simulink model "adc16_dbf_4fft"  (R2013a)
settings: Solver=ode45  StartTime=0.0  StopTime=2050  RelTol=1e-3
undefined symbols (not defined in the file): pfb_coeff_gen_calc
libraries: xbsIndex_r4 x1713, casper_library_misc x294, casper_library_delays x48, casper_library_pfbs x16, simulink x16, xps_library x1
(part 2 of 21)

== system adc16_dbf_4fft/gateway10 ==
  data[4] : Inport
  Bus Creator : BusCreator
  Bus Selector : BusSelector  OutputSignals=signal1,signal2,signal3,signal4
  Gateway Out{,1..3} (4 alike) : xbsIndex_r4/Gateway Out  inherit_from_input=off  hdl_port=on  timing_constraint=None  locs_specified=off  LOCs={}  UseAsDAC=off  DACChannel='1'  block_type=gatewayout
  to_scope : Outport
  wires:
  data[4]/1 -> Bus Selector/1
  Bus Selector/4 -> Gateway Out3/1  "<signal4>"
  Bus Selector/2 -> Gateway Out1/1  "<signal2>"
  Bus Selector/1 -> Gateway Out/1  "<signal1>"
  Bus Selector/3 -> Gateway Out2/1  "<signal3>"
  Bus Creator/1 -> to_scope/1
  Gateway Out/1 -> Bus Creator/1
  Gateway Out1/1 -> Bus Creator/2
  Gateway Out2/1 -> Bus Creator/3
  Gateway Out3/1 -> Bus Creator/4

== system adc16_dbf_4fft/gateway11 ==
  data[4] : Inport
  Bus Creator : BusCreator
  Bus Selector : BusSelector  OutputSignals=signal1,signal2,signal3,signal4
  Gateway Out{,1..3} (4 alike) : xbsIndex_r4/Gateway Out  inherit_from_input=off  hdl_port=on  timing_constraint=None  locs_specified=off  LOCs={}  UseAsDAC=off  DACChannel='1'  block_type=gatewayout
  to_scope : Outport
  wires:
  Gateway Out3/1 -> Bus Creator/4
  Gateway Out2/1 -> Bus Creator/3
  Gateway Out1/1 -> Bus Creator/2
  Gateway Out/1 -> Bus Creator/1
  Bus Creator/1 -> to_scope/1
  Bus Selector/3 -> Gateway Out2/1  "<signal3>"
  Bus Selector/1 -> Gateway Out/1  "<signal1>"
  Bus Selector/2 -> Gateway Out1/1  "<signal2>"
  Bus Selector/4 -> Gateway Out3/1  "<signal4>"
  data[4]/1 -> Bus Selector/1

== system adc16_dbf_4fft/gateway12 ==
  data[4] : Inport
  Bus Creator : BusCreator
  Bus Selector : BusSelector  OutputSignals=signal1,signal2,signal3,signal4
  Gateway Out{,1..3} (4 alike) : xbsIndex_r4/Gateway Out  inherit_from_input=off  hdl_port=on  timing_constraint=None  locs_specified=off  LOCs={}  UseAsDAC=off  DACChannel='1'  block_type=gatewayout
  to_scope : Outport
  wires:
  Gateway Out3/1 -> Bus Creator/4
  Gateway Out2/1 -> Bus Creator/3
  Gateway Out1/1 -> Bus Creator/2
  Gateway Out/1 -> Bus Creator/1
  Bus Creator/1 -> to_scope/1
  Bus Selector/3 -> Gateway Out2/1  "<signal3>"
  Bus Selector/1 -> Gateway Out/1  "<signal1>"
  Bus Selector/2 -> Gateway Out1/1  "<signal2>"
  Bus Selector/4 -> Gateway Out3/1  "<signal4>"
  data[4]/1 -> Bus Selector/1

== system adc16_dbf_4fft/gateway13 ==
  data[4] : Inport
  Bus Creator : BusCreator
  Bus Selector : BusSelector  OutputSignals=signal1,signal2,signal3,signal4
  Gateway Out{,1..3} (4 alike) : xbsIndex_r4/Gateway Out  inherit_from_input=off  hdl_port=on  timing_constraint=None  locs_specified=off  LOCs={}  UseAsDAC=off  DACChannel='1'  block_type=gatewayout
  to_scope : Outport
  wires:
  data[4]/1 -> Bus Selector/1
  Bus Selector/4 -> Gateway Out3/1  "<signal4>"
  Bus Selector/2 -> Gateway Out1/1  "<signal2>"
  Bus Selector/1 -> Gateway Out/1  "<signal1>"
  Bus Selector/3 -> Gateway Out2/1  "<signal3>"
  Bus Creator/1 -> to_scope/1
  Gateway Out/1 -> Bus Creator/1
  Gateway Out1/1 -> Bus Creator/2
  Gateway Out2/1 -> Bus Creator/3
  Gateway Out3/1 -> Bus Creator/4

== system adc16_dbf_4fft/gateway14 ==
  data[4] : Inport
  Bus Creator : BusCreator
  Bus Selector : BusSelector  OutputSignals=signal1,signal2,signal3,signal4
  Gateway Out{,1..3} (4 alike) : xbsIndex_r4/Gateway Out  inherit_from_input=off  hdl_port=on  timing_constraint=None  locs_specified=off  LOCs={}  UseAsDAC=off  DACChannel='1'  block_type=gatewayout
  to_scope : Outport
  wires:
  Gateway Out3/1 -> Bus Creator/4
  Gateway Out2/1 -> Bus Creator/3
  Gateway Out1/1 -> Bus Creator/2
  Gateway Out/1 -> Bus Creator/1
  Bus Creator/1 -> to_scope/1
  Bus Selector/3 -> Gateway Out2/1  "<signal3>"
  Bus Selector/1 -> Gateway Out/1  "<signal1>"
  Bus Selector/2 -> Gateway Out1/1  "<signal2>"
  Bus Selector/4 -> Gateway Out3/1  "<signal4>"
  data[4]/1 -> Bus Selector/1

== system adc16_dbf_4fft/gateway15 ==
  data[4] : Inport
  Bus Creator : BusCreator
  Bus Selector : BusSelector  OutputSignals=signal1,signal2,signal3,signal4
  Gateway Out{,1..3} (4 alike) : xbsIndex_r4/Gateway Out  inherit_from_input=off  hdl_port=on  timing_constraint=None  locs_specified=off  LOCs={}  UseAsDAC=off  DACChannel='1'  block_type=gatewayout
  to_scope : Outport
  wires:
  data[4]/1 -> Bus Selector/1
  Bus Selector/4 -> Gateway Out3/1  "<signal4>"
  Bus Selector/2 -> Gateway Out1/1  "<signal2>"
  Bus Selector/1 -> Gateway Out/1  "<signal1>"
  Bus Selector/3 -> Gateway Out2/1  "<signal3>"
  Bus Creator/1 -> to_scope/1
  Gateway Out/1 -> Bus Creator/1
  Gateway Out1/1 -> Bus Creator/2
  Gateway Out2/1 -> Bus Creator/3
  Gateway Out3/1 -> Bus Creator/4

== system adc16_dbf_4fft/gateway16 ==
  data[4] : Inport
  Bus Creator : BusCreator
  Bus Selector : BusSelector  OutputSignals=signal1,signal2,signal3,signal4
  Gateway Out{,1..3} (4 alike) : xbsIndex_r4/Gateway Out  inherit_from_input=off  hdl_port=on  timing_constraint=None  locs_specified=off  LOCs={}  UseAsDAC=off  DACChannel='1'  block_type=gatewayout
  to_scope : Outport
  wires:
  Gateway Out3/1 -> Bus Creator/4
  Gateway Out2/1 -> Bus Creator/3
  Gateway Out1/1 -> Bus Creator/2
  Gateway Out/1 -> Bus Creator/1
  Bus Creator/1 -> to_scope/1
  Bus Selector/3 -> Gateway Out2/1  "<signal3>"
  Bus Selector/1 -> Gateway Out/1  "<signal1>"
  Bus Selector/2 -> Gateway Out1/1  "<signal2>"
  Bus Selector/4 -> Gateway Out3/1  "<signal4>"
  data[4]/1 -> Bus Selector/1

== system adc16_dbf_4fft/gateway2 ==
  data[4] : Inport
  Bus Creator : BusCreator
  Bus Selector : BusSelector  OutputSignals=signal1,signal2,signal3,signal4
  Gateway Out{,1..3} (4 alike) : xbsIndex_r4/Gateway Out  inherit_from_input=off  hdl_port=on  timing_constraint=None  locs_specified=off  LOCs={}  UseAsDAC=off  DACChannel='1'  block_type=gatewayout
  to_scope : Outport
  wires:
  data[4]/1 -> Bus Selector/1
  Bus Selector/4 -> Gateway Out3/1  "<signal4>"
  Bus Selector/2 -> Gateway Out1/1  "<signal2>"
  Bus Selector/1 -> Gateway Out/1  "<signal1>"
  Bus Selector/3 -> Gateway Out2/1  "<signal3>"
  Bus Creator/1 -> to_scope/1
  Gateway Out/1 -> Bus Creator/1
  Gateway Out1/1 -> Bus Creator/2
  Gateway Out2/1 -> Bus Creator/3
  Gateway Out3/1 -> Bus Creator/4

== system adc16_dbf_4fft/gateway3 ==
  data[4] : Inport
  Bus Creator : BusCreator
  Bus Selector : BusSelector  OutputSignals=signal1,signal2,signal3,signal4
  Gateway Out{,1..3} (4 alike) : xbsIndex_r4/Gateway Out  inherit_from_input=off  hdl_port=on  timing_constraint=None  locs_specified=off  LOCs={}  UseAsDAC=off  DACChannel='1'  block_type=gatewayout
  to_scope : Outport
  wires:
  data[4]/1 -> Bus Selector/1
  Bus Selector/4 -> Gateway Out3/1  "<signal4>"
  Bus Selector/2 -> Gateway Out1/1  "<signal2>"
  Bus Selector/1 -> Gateway Out/1  "<signal1>"
  Bus Selector/3 -> Gateway Out2/1  "<signal3>"
  Bus Creator/1 -> to_scope/1
  Gateway Out/1 -> Bus Creator/1
  Gateway Out1/1 -> Bus Creator/2
  Gateway Out2/1 -> Bus Creator/3
  Gateway Out3/1 -> Bus Creator/4

== system adc16_dbf_4fft/gateway4 ==
  data[4] : Inport
  Bus Creator : BusCreator
  Bus Selector : BusSelector  OutputSignals=signal1,signal2,signal3,signal4
  Gateway Out{,1..3} (4 alike) : xbsIndex_r4/Gateway Out  inherit_from_input=off  hdl_port=on  timing_constraint=None  locs_specified=off  LOCs={}  UseAsDAC=off  DACChannel='1'  block_type=gatewayout
  to_scope : Outport
  wires:
  Gateway Out3/1 -> Bus Creator/4
  Gateway Out2/1 -> Bus Creator/3
  Gateway Out1/1 -> Bus Creator/2
  Gateway Out/1 -> Bus Creator/1
  Bus Creator/1 -> to_scope/1
  Bus Selector/3 -> Gateway Out2/1  "<signal3>"
  Bus Selector/1 -> Gateway Out/1  "<signal1>"
  Bus Selector/2 -> Gateway Out1/1  "<signal2>"
  Bus Selector/4 -> Gateway Out3/1  "<signal4>"
  data[4]/1 -> Bus Selector/1

== system adc16_dbf_4fft/gateway5 ==
  data[4] : Inport
  Bus Creator : BusCreator
  Bus Selector : BusSelector  OutputSignals=signal1,signal2,signal3,signal4
  Gateway Out{,1..3} (4 alike) : xbsIndex_r4/Gateway Out  inherit_from_input=off  hdl_port=on  timing_constraint=None  locs_specified=off  LOCs={}  UseAsDAC=off  DACChannel='1'  block_type=gatewayout
  to_scope : Outport
  wires:
  data[4]/1 -> Bus Selector/1
  Bus Selector/4 -> Gateway Out3/1  "<signal4>"
  Bus Selector/2 -> Gateway Out1/1  "<signal2>"
  Bus Selector/1 -> Gateway Out/1  "<signal1>"
  Bus Selector/3 -> Gateway Out2/1  "<signal3>"
  Bus Creator/1 -> to_scope/1
  Gateway Out/1 -> Bus Creator/1
  Gateway Out1/1 -> Bus Creator/2
  Gateway Out2/1 -> Bus Creator/3
  Gateway Out3/1 -> Bus Creator/4

== system adc16_dbf_4fft/gateway6 ==
  data[4] : Inport
  Bus Creator : BusCreator
  Bus Selector : BusSelector  OutputSignals=signal1,signal2,signal3,signal4
  Gateway Out{,1..3} (4 alike) : xbsIndex_r4/Gateway Out  inherit_from_input=off  hdl_port=on  timing_constraint=None  locs_specified=off  LOCs={}  UseAsDAC=off  DACChannel='1'  block_type=gatewayout
  to_scope : Outport
  wires:
  data[4]/1 -> Bus Selector/1
  Bus Selector/4 -> Gateway Out3/1  "<signal4>"
  Bus Selector/2 -> Gateway Out1/1  "<signal2>"
  Bus Selector/1 -> Gateway Out/1  "<signal1>"
  Bus Selector/3 -> Gateway Out2/1  "<signal3>"
  Bus Creator/1 -> to_scope/1
  Gateway Out/1 -> Bus Creator/1
  Gateway Out1/1 -> Bus Creator/2
  Gateway Out2/1 -> Bus Creator/3
  Gateway Out3/1 -> Bus Creator/4

== system adc16_dbf_4fft/gateway7 ==
  data[4] : Inport
  Bus Creator : BusCreator
  Bus Selector : BusSelector  OutputSignals=signal1,signal2,signal3,signal4
  Gateway Out{,1..3} (4 alike) : xbsIndex_r4/Gateway Out  inherit_from_input=off  hdl_port=on  timing_constraint=None  locs_specified=off  LOCs={}  UseAsDAC=off  DACChannel='1'  block_type=gatewayout
  to_scope : Outport
  wires:
  Gateway Out3/1 -> Bus Creator/4
  Gateway Out2/1 -> Bus Creator/3
  Gateway Out1/1 -> Bus Creator/2
  Gateway Out/1 -> Bus Creator/1
  Bus Creator/1 -> to_scope/1
  Bus Selector/3 -> Gateway Out2/1  "<signal3>"
  Bus Selector/1 -> Gateway Out/1  "<signal1>"
  Bus Selector/2 -> Gateway Out1/1  "<signal2>"
  Bus Selector/4 -> Gateway Out3/1  "<signal4>"
  data[4]/1 -> Bus Selector/1

== system adc16_dbf_4fft/gateway8 ==
  data[4] : Inport
  Bus Creator : BusCreator
  Bus Selector : BusSelector  OutputSignals=signal1,signal2,signal3,signal4
  Gateway Out{,1..3} (4 alike) : xbsIndex_r4/Gateway Out  inherit_from_input=off  hdl_port=on  timing_constraint=None  locs_specified=off  LOCs={}  UseAsDAC=off  DACChannel='1'  block_type=gatewayout
  to_scope : Outport
  wires:
  Gateway Out3/1 -> Bus Creator/4
  Gateway Out2/1 -> Bus Creator/3
  Gateway Out1/1 -> Bus Creator/2
  Gateway Out/1 -> Bus Creator/1
  Bus Creator/1 -> to_scope/1
  Bus Selector/3 -> Gateway Out2/1  "<signal3>"
  Bus Selector/1 -> Gateway Out/1  "<signal1>"
  Bus Selector/2 -> Gateway Out1/1  "<signal2>"
  Bus Selector/4 -> Gateway Out3/1  "<signal4>"
  data[4]/1 -> Bus Selector/1

== system adc16_dbf_4fft/gateway9 ==
  data[4] : Inport
  Bus Creator : BusCreator
  Bus Selector : BusSelector  OutputSignals=signal1,signal2,signal3,signal4
  Gateway Out{,1..3} (4 alike) : xbsIndex_r4/Gateway Out  inherit_from_input=off  hdl_port=on  timing_constraint=None  locs_specified=off  LOCs={}  UseAsDAC=off  DACChannel='1'  block_type=gatewayout
  to_scope : Outport
  wires:
  data[4]/1 -> Bus Selector/1
  Bus Selector/4 -> Gateway Out3/1  "<signal4>"
  Bus Selector/2 -> Gateway Out1/1  "<signal2>"
  Bus Selector/1 -> Gateway Out/1  "<signal1>"
  Bus Selector/3 -> Gateway Out2/1  "<signal3>"
  Bus Creator/1 -> to_scope/1
  Gateway Out/1 -> Bus Creator/1
  Gateway Out1/1 -> Bus Creator/2
  Gateway Out2/1 -> Bus Creator/3
  Gateway Out3/1 -> Bus Creator/4

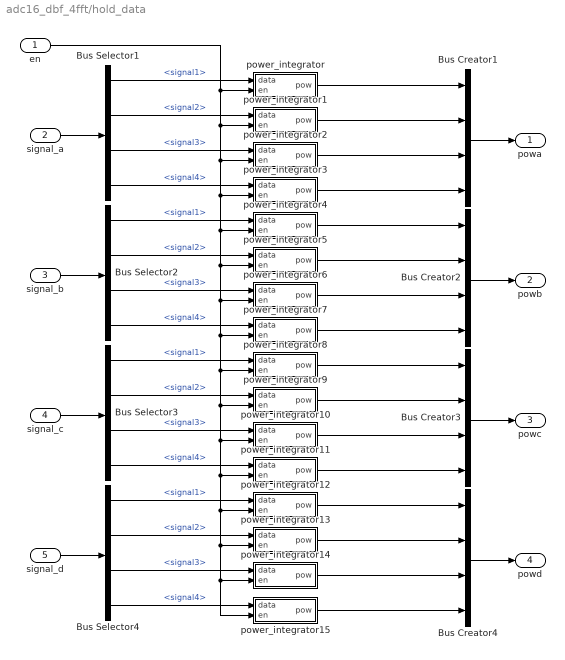
== system adc16_dbf_4fft/hold_data ==
  en : Inport
  signal_a : Inport  Port=2
  signal_b : Inport  Port=3
  signal_c : Inport  Port=4
  signal_d : Inport  Port=5
  Bus Creator{1..4} (4 alike) : BusCreator
  Bus Selector{1..4} (4 alike) : BusSelector  OutputSignals=signal1,signal2,signal3,signal4
  power_integrator : Subsystem
  power_integrator1 : Subsystem
  power_integrator10 : Subsystem
  power_integrator11 : Subsystem
  power_integrator12 : Subsystem
  power_integrator13 : Subsystem
  power_integrator14 : Subsystem
  power_integrator15 : Subsystem
  power_integrator2 : Subsystem
  power_integrator3 : Subsystem
  power_integrator4 : Subsystem
  power_integrator5 : Subsystem
  power_integrator6 : Subsystem
  power_integrator7 : Subsystem
  power_integrator8 : Subsystem
  power_integrator9 : Subsystem
  powa : Outport
  powb : Outport  Port=2
  powc : Outport  Port=3
  powd : Outport  Port=4
  wires:
  power_integrator4/1(pow) -> Bus Creator2/1
  power_integrator1/1(pow) -> Bus Creator1/2
  power_integrator5/1(pow) -> Bus Creator2/2
  power_integrator6/1(pow) -> Bus Creator2/3
  power_integrator2/1(pow) -> Bus Creator1/3
  power_integrator7/1(pow) -> Bus Creator2/4
  power_integrator3/1(pow) -> Bus Creator1/4
  Bus Creator1/1 -> powa/1
  power_integrator/1(pow) -> Bus Creator1/1
  power_integrator11/1(pow) -> Bus Creator3/4
  power_integrator8/1(pow) -> Bus Creator3/1
  power_integrator14/1(pow) -> Bus Creator4/3
  power_integrator12/1(pow) -> Bus Creator4/1
  power_integrator15/1(pow) -> Bus Creator4/4
  power_integrator10/1(pow) -> Bus Creator3/3
  power_integrator9/1(pow) -> Bus Creator3/2
  power_integrator13/1(pow) -> Bus Creator4/2
  en/1 -> power_integrator15/2(en), power_integrator14/2(en), power_integrator13/2(en), power_integrator12/2(en), power_integrator11/2(en), power_integrator10/2(en), power_integrator9/2(en), power_integrator8/2(en), power_integrator7/2(en), power_integrator6/2(en), power_integrator5/2(en), power_integrator4/2(en), power_integrator3/2(en), power_integrator2/2(en), power_integrator1/2(en), power_integrator/2(en)
  signal_a/1 -> Bus Selector1/1
  signal_d/1 -> Bus Selector4/1
  signal_c/1 -> Bus Selector3/1
  Bus Selector1/1 -> power_integrator/1(data)  "<signal1>"
  Bus Selector1/2 -> power_integrator1/1(data)  "<signal2>"
  Bus Selector1/3 -> power_integrator2/1(data)  "<signal3>"
  Bus Selector1/4 -> power_integrator3/1(data)  "<signal4>"
  signal_b/1 -> Bus Selector2/1
  Bus Selector2/1 -> power_integrator4/1(data)  "<signal1>"
  Bus Selector2/2 -> power_integrator5/1(data)  "<signal2>"
  Bus Selector2/3 -> power_integrator6/1(data)  "<signal3>"
  Bus Selector2/4 -> power_integrator7/1(data)  "<signal4>"
  Bus Selector3/1 -> power_integrator8/1(data)  "<signal1>"
  Bus Selector3/2 -> power_integrator9/1(data)  "<signal2>"
  Bus Selector3/3 -> power_integrator10/1(data)  "<signal3>"
  Bus Selector3/4 -> power_integrator11/1(data)  "<signal4>"
  Bus Selector4/1 -> power_integrator12/1(data)  "<signal1>"
  Bus Selector4/2 -> power_integrator13/1(data)  "<signal2>"
  Bus Selector4/3 -> power_integrator14/1(data)  "<signal3>"
  Bus Selector4/4 -> power_integrator15/1(data)  "<signal4>"
  Bus Creator4/1 -> powd/1
  Bus Creator3/1 -> powc/1
  Bus Creator2/1 -> powb/1

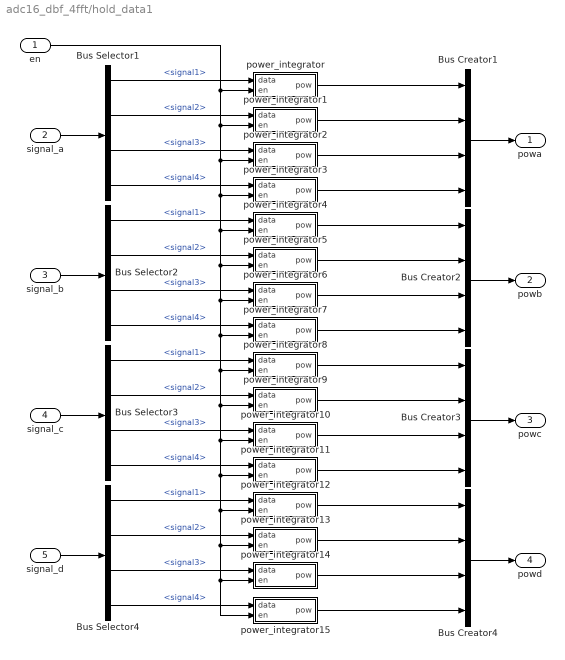
== system adc16_dbf_4fft/hold_data1 ==
  en : Inport
  signal_a : Inport  Port=2
  signal_b : Inport  Port=3
  signal_c : Inport  Port=4
  signal_d : Inport  Port=5
  Bus Creator{1..4} (4 alike) : BusCreator
  Bus Selector{1..4} (4 alike) : BusSelector  OutputSignals=signal1,signal2,signal3,signal4
  power_integrator : Subsystem
  power_integrator1 : Subsystem
  power_integrator10 : Subsystem
  power_integrator11 : Subsystem
  power_integrator12 : Subsystem
  power_integrator13 : Subsystem
  power_integrator14 : Subsystem
  power_integrator15 : Subsystem
  power_integrator2 : Subsystem
  power_integrator3 : Subsystem
  power_integrator4 : Subsystem
  power_integrator5 : Subsystem
  power_integrator6 : Subsystem
  power_integrator7 : Subsystem
  power_integrator8 : Subsystem
  power_integrator9 : Subsystem
  powa : Outport
  powb : Outport  Port=2
  powc : Outport  Port=3
  powd : Outport  Port=4
  wires:
  Bus Creator2/1 -> powb/1
  Bus Creator3/1 -> powc/1
  Bus Creator4/1 -> powd/1
  Bus Selector4/4 -> power_integrator15/1(data)  "<signal4>"
  Bus Selector4/3 -> power_integrator14/1(data)  "<signal3>"
  Bus Selector4/2 -> power_integrator13/1(data)  "<signal2>"
  Bus Selector4/1 -> power_integrator12/1(data)  "<signal1>"
  Bus Selector3/4 -> power_integrator11/1(data)  "<signal4>"
  Bus Selector3/3 -> power_integrator10/1(data)  "<signal3>"
  Bus Selector3/2 -> power_integrator9/1(data)  "<signal2>"
  Bus Selector3/1 -> power_integrator8/1(data)  "<signal1>"
  Bus Selector2/4 -> power_integrator7/1(data)  "<signal4>"
  Bus Selector2/3 -> power_integrator6/1(data)  "<signal3>"
  Bus Selector2/2 -> power_integrator5/1(data)  "<signal2>"
  Bus Selector2/1 -> power_integrator4/1(data)  "<signal1>"
  signal_b/1 -> Bus Selector2/1
  Bus Selector1/4 -> power_integrator3/1(data)  "<signal4>"
  Bus Selector1/3 -> power_integrator2/1(data)  "<signal3>"
  Bus Selector1/2 -> power_integrator1/1(data)  "<signal2>"
  Bus Selector1/1 -> power_integrator/1(data)  "<signal1>"
  signal_c/1 -> Bus Selector3/1
  signal_d/1 -> Bus Selector4/1
  signal_a/1 -> Bus Selector1/1
  en/1 -> power_integrator/2(en), power_integrator1/2(en), power_integrator2/2(en), power_integrator3/2(en), power_integrator4/2(en), power_integrator5/2(en), power_integrator6/2(en), power_integrator7/2(en), power_integrator8/2(en), power_integrator9/2(en), power_integrator10/2(en), power_integrator11/2(en), power_integrator12/2(en), power_integrator13/2(en), power_integrator14/2(en), power_integrator15/2(en)
  power_integrator13/1(pow) -> Bus Creator4/2
  power_integrator9/1(pow) -> Bus Creator3/2
  power_integrator10/1(pow) -> Bus Creator3/3
  power_integrator15/1(pow) -> Bus Creator4/4
  power_integrator12/1(pow) -> Bus Creator4/1
  power_integrator14/1(pow) -> Bus Creator4/3
  power_integrator8/1(pow) -> Bus Creator3/1
  power_integrator11/1(pow) -> Bus Creator3/4
  power_integrator/1(pow) -> Bus Creator1/1
  Bus Creator1/1 -> powa/1
  power_integrator3/1(pow) -> Bus Creator1/4
  power_integrator7/1(pow) -> Bus Creator2/4
  power_integrator2/1(pow) -> Bus Creator1/3
  power_integrator6/1(pow) -> Bus Creator2/3
  power_integrator5/1(pow) -> Bus Creator2/2
  power_integrator1/1(pow) -> Bus Creator1/2
  power_integrator4/1(pow) -> Bus Creator2/1

== system adc16_dbf_4fft/pfb_single_channel ==
  sync : Inport
  pol1_in : Inport  Port=2
  pol2_in : Inport  Port=3
  pol3_in : Inport  Port=4
  pol4_in : Inport  Port=5
  Terminator : Terminator
  Terminator1 : Terminator
  Terminator2 : Terminator
  pfb_fir_real1 : Subsystem  Tag=casper:pfb_fir_real  AncestorBlock=casper_library_pfbs/pfb_fir_real  mask(pfb_fir_real){PFBSize=2, TotalTaps=4, WindowType=hamming, n_inputs=0, MakeBiplex=off, BitWidthIn=8, BitWidthOut=18, CoeffBitWidth=18, CoeffDistMem=off, add_latency=1, mult_latency=2, bram_latency=2, fan_latency=1, conv_latency=1, quantization=Round  (unbiased: Even Values), fwidth=1, mult_spec=2, adder_folding=on, adder_imp=Fabric, coeffs_share=off}
      mask prompts: PFBSize "Size of PFB: (2^? pnts)"; TotalTaps "Total Number of Taps:"; WindowType "Windowing Function:"; n_inputs "Number of Simultaneous Inputs: (2^?)"; MakeBiplex "Make Biplex?"; BitWidthIn "Input Bitwidth:"; BitWidthOut "Output Bitwidth:"; CoeffBitWidth "Coefficient Bitwidth:"; CoeffDistMem "Use Distributed Memory for Coeffs"; add_latency "Add Latency"; mult_latency "Mult Latency"; bram_latency "BRAM Latency"; fan_latency "Fanout latency"; conv_latency "Convert latency"; quantization "Quantization Behavior"; fwidth "Bin Width Scaling (normal=1)"; mult_spec "Multiplier specification (0=core, 1=embedded, 2=behavioural) (left=1st tap, or just one value)"; adder_folding "Fold adders into DSPs"; adder_imp "Adder implementation"; coeffs_share "Share coefficients between polarisations (use less BRAM)?"
      mask help:
      | Fold adders into DSPs: Causes adders to be absorbed into DSP blocks (supported in Virtex5)
      | Adder implementation: Cores using Fabric or DSP48 or behavioral HDL
      mask init:
      | pfb_fir_real_init(gcb, ...
      |     'PFBSize', PFBSize, ...
      |     'TotalTaps', TotalTaps, ...
      |     'WindowType', WindowType, ...
      |     'n_inputs', n_inputs, ...
      |     'MakeBiplex', MakeBiplex, ...
      |     'BitWidthIn', BitWidthIn, ...
      |     'BitWidthOut', BitWidthOut, ...
      |     'CoeffBitWidth', CoeffBitWidth, ...
      |     'CoeffDistMem', CoeffDistMem, ...
      |     'add_latency', add_latency, ...
      |     'mult_latency', mult_latency, ...
      |     'bram_latency', bram_latency, ...
      |     'fan_latency', fan_latency, ...
      |     'conv_latency', conv_latency, ...
      |     'quantization', quantization, ...
      |     'fwidth', fwidth, ...
      |     'mult_spec', mult_spec, ...
      |     'adder_folding', adder_folding, ...
      |     'adder_imp', adder_imp, ...
      |     'coeffs_share', coeffs_share);
      settings: AttributesFormatString=taps=4, add_latency=1
      mask Help: eval('xlWeb(''http://casper.berkeley.edu/wiki/Pfb_fir_real'')')
      mask Callback TotalTaps:
      | %num_taps = eval(get_param(gcb, 'TotalTaps'));
      | %old_vec = eval(get_param(gcb, 'mult_spec'));=-0l
      | 
      | %vec = 2.*ones(1,num_taps);
      | %old_size = length(old_vec);
      | 
      | %if(old_size <= num_taps),
      | %    new_size = old_size;
      | %else,
      | %    new_size = num_taps;
      | %end
      | 
      | %for n = 1:new_size, vec(n) = old_vec(n); end
      | %set_param(gcb, 'mult_spec', mat2str(vec));
      mask TypeOptions WindowType: bartlett | barthannwin | blackman | blackmanharris | bohamwin | chebwin | flattopwin | gausswin | hamming | hann | kaiser | nuttallwin | parzenwin | rectwin | tukeywin | triang | userwindow
      mask TypeOptions quantization: Truncate | Round  (unbiased: +/- Inf) | Round  (unbiased: Even Values)
      mask TypeOptions adder_imp: Behavioral | Fabric | DSP48
  pfb_fir_real2 : Subsystem  Tag=casper:pfb_fir_real  AncestorBlock=casper_library_pfbs/pfb_fir_real  mask(pfb_fir_real){PFBSize=2, TotalTaps=4, WindowType=hamming, n_inputs=0, MakeBiplex=off, BitWidthIn=8, BitWidthOut=18, CoeffBitWidth=18, CoeffDistMem=off, add_latency=1, mult_latency=2, bram_latency=2, fan_latency=1, conv_latency=1, quantization=Round  (unbiased: Even Values), fwidth=1, mult_spec=2, adder_folding=on, adder_imp=Fabric, coeffs_share=off}
      mask prompts: PFBSize "Size of PFB: (2^? pnts)"; TotalTaps "Total Number of Taps:"; WindowType "Windowing Function:"; n_inputs "Number of Simultaneous Inputs: (2^?)"; MakeBiplex "Make Biplex?"; BitWidthIn "Input Bitwidth:"; BitWidthOut "Output Bitwidth:"; CoeffBitWidth "Coefficient Bitwidth:"; CoeffDistMem "Use Distributed Memory for Coeffs"; add_latency "Add Latency"; mult_latency "Mult Latency"; bram_latency "BRAM Latency"; fan_latency "Fanout latency"; conv_latency "Convert latency"; quantization "Quantization Behavior"; fwidth "Bin Width Scaling (normal=1)"; mult_spec "Multiplier specification (0=core, 1=embedded, 2=behavioural) (left=1st tap, or just one value)"; adder_folding "Fold adders into DSPs"; adder_imp "Adder implementation"; coeffs_share "Share coefficients between polarisations (use less BRAM)?"
      mask help:
      | Fold adders into DSPs: Causes adders to be absorbed into DSP blocks (supported in Virtex5)
      | Adder implementation: Cores using Fabric or DSP48 or behavioral HDL
      mask init: same as adc16_dbf_4fft/pfb_single_channel/pfb_fir_real1
      settings: AttributesFormatString=taps=4, add_latency=1
      mask Help: eval('xlWeb(''http://casper.berkeley.edu/wiki/Pfb_fir_real'')')
      mask Callback TotalTaps:
      | %num_taps = eval(get_param(gcb, 'TotalTaps'));
      | %old_vec = eval(get_param(gcb, 'mult_spec'));=-0l
      | 
      | %vec = 2.*ones(1,num_taps);
      | %old_size = length(old_vec);
      | 
      | %if(old_size <= num_taps),
      | %    new_size = old_size;
      | %else,
      | %    new_size = num_taps;
      | %end
      | 
      | %for n = 1:new_size, vec(n) = old_vec(n); end
      | %set_param(gcb, 'mult_spec', mat2str(vec));
      mask TypeOptions WindowType: bartlett | barthannwin | blackman | blackmanharris | bohamwin | chebwin | flattopwin | gausswin | hamming | hann | kaiser | nuttallwin | parzenwin | rectwin | tukeywin | triang | userwindow
      mask TypeOptions quantization: Truncate | Round  (unbiased: +/- Inf) | Round  (unbiased: Even Values)
      mask TypeOptions adder_imp: Behavioral | Fabric | DSP48
  pfb_fir_real3 : Subsystem  Tag=casper:pfb_fir_real  AncestorBlock=casper_library_pfbs/pfb_fir_real  mask(pfb_fir_real){PFBSize=2, TotalTaps=4, WindowType=hamming, n_inputs=0, MakeBiplex=off, BitWidthIn=8, BitWidthOut=18, CoeffBitWidth=18, CoeffDistMem=off, add_latency=1, mult_latency=2, bram_latency=2, fan_latency=1, conv_latency=1, quantization=Round  (unbiased: Even Values), fwidth=1, mult_spec=2, adder_folding=on, adder_imp=Fabric, coeffs_share=off}
      mask prompts: PFBSize "Size of PFB: (2^? pnts)"; TotalTaps "Total Number of Taps:"; WindowType "Windowing Function:"; n_inputs "Number of Simultaneous Inputs: (2^?)"; MakeBiplex "Make Biplex?"; BitWidthIn "Input Bitwidth:"; BitWidthOut "Output Bitwidth:"; CoeffBitWidth "Coefficient Bitwidth:"; CoeffDistMem "Use Distributed Memory for Coeffs"; add_latency "Add Latency"; mult_latency "Mult Latency"; bram_latency "BRAM Latency"; fan_latency "Fanout latency"; conv_latency "Convert latency"; quantization "Quantization Behavior"; fwidth "Bin Width Scaling (normal=1)"; mult_spec "Multiplier specification (0=core, 1=embedded, 2=behavioural) (left=1st tap, or just one value)"; adder_folding "Fold adders into DSPs"; adder_imp "Adder implementation"; coeffs_share "Share coefficients between polarisations (use less BRAM)?"
      mask help:
      | Fold adders into DSPs: Causes adders to be absorbed into DSP blocks (supported in Virtex5)
      | Adder implementation: Cores using Fabric or DSP48 or behavioral HDL
      mask init: same as adc16_dbf_4fft/pfb_single_channel/pfb_fir_real1
      settings: AttributesFormatString=taps=4, add_latency=1
      mask Help: eval('xlWeb(''http://casper.berkeley.edu/wiki/Pfb_fir_real'')')
      mask Callback TotalTaps:
      | %num_taps = eval(get_param(gcb, 'TotalTaps'));
      | %old_vec = eval(get_param(gcb, 'mult_spec'));=-0l
      | 
      | %vec = 2.*ones(1,num_taps);
      | %old_size = length(old_vec);
      | 
      | %if(old_size <= num_taps),
      | %    new_size = old_size;
      | %else,
      | %    new_size = num_taps;
      | %end
      | 
      | %for n = 1:new_size, vec(n) = old_vec(n); end
      | %set_param(gcb, 'mult_spec', mat2str(vec));
      mask TypeOptions WindowType: bartlett | barthannwin | blackman | blackmanharris | bohamwin | chebwin | flattopwin | gausswin | hamming | hann | kaiser | nuttallwin | parzenwin | rectwin | tukeywin | triang | userwindow
      mask TypeOptions quantization: Truncate | Round  (unbiased: +/- Inf) | Round  (unbiased: Even Values)
      mask TypeOptions adder_imp: Behavioral | Fabric | DSP48
  pfb_fir_real4 : Subsystem  Tag=casper:pfb_fir_real  AncestorBlock=casper_library_pfbs/pfb_fir_real  mask(pfb_fir_real){PFBSize=2, TotalTaps=4, WindowType=hamming, n_inputs=0, MakeBiplex=off, BitWidthIn=8, BitWidthOut=18, CoeffBitWidth=18, CoeffDistMem=off, add_latency=1, mult_latency=2, bram_latency=2, fan_latency=1, conv_latency=1, quantization=Round  (unbiased: Even Values), fwidth=1, mult_spec=2, adder_folding=on, adder_imp=Fabric, coeffs_share=off}
      mask prompts: PFBSize "Size of PFB: (2^? pnts)"; TotalTaps "Total Number of Taps:"; WindowType "Windowing Function:"; n_inputs "Number of Simultaneous Inputs: (2^?)"; MakeBiplex "Make Biplex?"; BitWidthIn "Input Bitwidth:"; BitWidthOut "Output Bitwidth:"; CoeffBitWidth "Coefficient Bitwidth:"; CoeffDistMem "Use Distributed Memory for Coeffs"; add_latency "Add Latency"; mult_latency "Mult Latency"; bram_latency "BRAM Latency"; fan_latency "Fanout latency"; conv_latency "Convert latency"; quantization "Quantization Behavior"; fwidth "Bin Width Scaling (normal=1)"; mult_spec "Multiplier specification (0=core, 1=embedded, 2=behavioural) (left=1st tap, or just one value)"; adder_folding "Fold adders into DSPs"; adder_imp "Adder implementation"; coeffs_share "Share coefficients between polarisations (use less BRAM)?"
      mask help:
      | Fold adders into DSPs: Causes adders to be absorbed into DSP blocks (supported in Virtex5)
      | Adder implementation: Cores using Fabric or DSP48 or behavioral HDL
      mask init: same as adc16_dbf_4fft/pfb_single_channel/pfb_fir_real1
      settings: AttributesFormatString=taps=4, add_latency=1
      mask Help: eval('xlWeb(''http://casper.berkeley.edu/wiki/Pfb_fir_real'')')
      mask Callback TotalTaps:
      | %num_taps = eval(get_param(gcb, 'TotalTaps'));
      | %old_vec = eval(get_param(gcb, 'mult_spec'));=-0l
      | 
      | %vec = 2.*ones(1,num_taps);
      | %old_size = length(old_vec);
      | 
      | %if(old_size <= num_taps),
      | %    new_size = old_size;
      | %else,
      | %    new_size = num_taps;
      | %end
      | 
      | %for n = 1:new_size, vec(n) = old_vec(n); end
      | %set_param(gcb, 'mult_spec', mat2str(vec));
      mask TypeOptions WindowType: bartlett | barthannwin | blackman | blackmanharris | bohamwin | chebwin | flattopwin | gausswin | hamming | hann | kaiser | nuttallwin | parzenwin | rectwin | tukeywin | triang | userwindow
      mask TypeOptions quantization: Truncate | Round  (unbiased: +/- Inf) | Round  (unbiased: Even Values)
      mask TypeOptions adder_imp: Behavioral | Fabric | DSP48
  sync_out : Outport
  pol1_out : Outport  Port=2
  pol2_out : Outport  Port=3
  pol3_out : Outport  Port=4
  pol4_out : Outport  Port=5
  wires:
  pol2_in/1 -> pfb_fir_real2/2(pol1_in1)
  pol3_in/1 -> pfb_fir_real3/2(pol1_in1)
  pfb_fir_real1/2(pol1_out1) -> pol1_out/1
  sync/1 -> pfb_fir_real4/1(sync), pfb_fir_real3/1(sync), pfb_fir_real2/1(sync), pfb_fir_real1/1(sync)
  pfb_fir_real3/2(pol1_out1) -> pol3_out/1
  pfb_fir_real4/2(pol1_out1) -> pol4_out/1
  pol1_in/1 -> pfb_fir_real1/2(pol1_in1)
  pol4_in/1 -> pfb_fir_real4/2(pol1_in1)
  pfb_fir_real2/2(pol1_out1) -> pol2_out/1
  pfb_fir_real1/1(sync_out) -> sync_out/1
  pfb_fir_real2/1(sync_out) -> Terminator/1
  pfb_fir_real3/1(sync_out) -> Terminator1/1
  pfb_fir_real4/1(sync_out) -> Terminator2/1

== system adc16_dbf_4fft/pfb_single_channel1 ==
  sync : Inport
  pol1_in : Inport  Port=2
  pol2_in : Inport  Port=3
  pol3_in : Inport  Port=4
  pol4_in : Inport  Port=5
  Terminator : Terminator
  Terminator1 : Terminator
  Terminator2 : Terminator
  pfb_fir_real1 : Subsystem  Tag=casper:pfb_fir_real  AncestorBlock=casper_library_pfbs/pfb_fir_real  mask(pfb_fir_real){PFBSize=2, TotalTaps=4, WindowType=hamming, n_inputs=0, MakeBiplex=off, BitWidthIn=8, BitWidthOut=18, CoeffBitWidth=18, CoeffDistMem=off, add_latency=1, mult_latency=2, bram_latency=2, fan_latency=1, conv_latency=1, quantization=Round  (unbiased: Even Values), fwidth=1, mult_spec=2, adder_folding=on, adder_imp=Fabric, coeffs_share=off}
      mask prompts: PFBSize "Size of PFB: (2^? pnts)"; TotalTaps "Total Number of Taps:"; WindowType "Windowing Function:"; n_inputs "Number of Simultaneous Inputs: (2^?)"; MakeBiplex "Make Biplex?"; BitWidthIn "Input Bitwidth:"; BitWidthOut "Output Bitwidth:"; CoeffBitWidth "Coefficient Bitwidth:"; CoeffDistMem "Use Distributed Memory for Coeffs"; add_latency "Add Latency"; mult_latency "Mult Latency"; bram_latency "BRAM Latency"; fan_latency "Fanout latency"; conv_latency "Convert latency"; quantization "Quantization Behavior"; fwidth "Bin Width Scaling (normal=1)"; mult_spec "Multiplier specification (0=core, 1=embedded, 2=behavioural) (left=1st tap, or just one value)"; adder_folding "Fold adders into DSPs"; adder_imp "Adder implementation"; coeffs_share "Share coefficients between polarisations (use less BRAM)?"
      mask help:
      | Fold adders into DSPs: Causes adders to be absorbed into DSP blocks (supported in Virtex5)
      | Adder implementation: Cores using Fabric or DSP48 or behavioral HDL
      mask init: same as adc16_dbf_4fft/pfb_single_channel/pfb_fir_real1
      settings: AttributesFormatString=taps=4, add_latency=1
      mask Help: eval('xlWeb(''http://casper.berkeley.edu/wiki/Pfb_fir_real'')')
      mask Callback TotalTaps:
      | %num_taps = eval(get_param(gcb, 'TotalTaps'));
      | %old_vec = eval(get_param(gcb, 'mult_spec'));=-0l
      | 
      | %vec = 2.*ones(1,num_taps);
      | %old_size = length(old_vec);
      | 
      | %if(old_size <= num_taps),
      | %    new_size = old_size;
      | %else,
      | %    new_size = num_taps;
      | %end
      | 
      | %for n = 1:new_size, vec(n) = old_vec(n); end
      | %set_param(gcb, 'mult_spec', mat2str(vec));
      mask TypeOptions WindowType: bartlett | barthannwin | blackman | blackmanharris | bohamwin | chebwin | flattopwin | gausswin | hamming | hann | kaiser | nuttallwin | parzenwin | rectwin | tukeywin | triang | userwindow
      mask TypeOptions quantization: Truncate | Round  (unbiased: +/- Inf) | Round  (unbiased: Even Values)
      mask TypeOptions adder_imp: Behavioral | Fabric | DSP48
  pfb_fir_real2 : Subsystem  Tag=casper:pfb_fir_real  AncestorBlock=casper_library_pfbs/pfb_fir_real  mask(pfb_fir_real){PFBSize=2, TotalTaps=4, WindowType=hamming, n_inputs=0, MakeBiplex=off, BitWidthIn=8, BitWidthOut=18, CoeffBitWidth=18, CoeffDistMem=off, add_latency=1, mult_latency=2, bram_latency=2, fan_latency=1, conv_latency=1, quantization=Round  (unbiased: Even Values), fwidth=1, mult_spec=2, adder_folding=on, adder_imp=Fabric, coeffs_share=off}
      mask prompts: PFBSize "Size of PFB: (2^? pnts)"; TotalTaps "Total Number of Taps:"; WindowType "Windowing Function:"; n_inputs "Number of Simultaneous Inputs: (2^?)"; MakeBiplex "Make Biplex?"; BitWidthIn "Input Bitwidth:"; BitWidthOut "Output Bitwidth:"; CoeffBitWidth "Coefficient Bitwidth:"; CoeffDistMem "Use Distributed Memory for Coeffs"; add_latency "Add Latency"; mult_latency "Mult Latency"; bram_latency "BRAM Latency"; fan_latency "Fanout latency"; conv_latency "Convert latency"; quantization "Quantization Behavior"; fwidth "Bin Width Scaling (normal=1)"; mult_spec "Multiplier specification (0=core, 1=embedded, 2=behavioural) (left=1st tap, or just one value)"; adder_folding "Fold adders into DSPs"; adder_imp "Adder implementation"; coeffs_share "Share coefficients between polarisations (use less BRAM)?"
      mask help:
      | Fold adders into DSPs: Causes adders to be absorbed into DSP blocks (supported in Virtex5)
      | Adder implementation: Cores using Fabric or DSP48 or behavioral HDL
      mask init: same as adc16_dbf_4fft/pfb_single_channel/pfb_fir_real1
      settings: AttributesFormatString=taps=4, add_latency=1
      mask Help: eval('xlWeb(''http://casper.berkeley.edu/wiki/Pfb_fir_real'')')
      mask Callback TotalTaps:
      | %num_taps = eval(get_param(gcb, 'TotalTaps'));
      | %old_vec = eval(get_param(gcb, 'mult_spec'));=-0l
      | 
      | %vec = 2.*ones(1,num_taps);
      | %old_size = length(old_vec);
      | 
      | %if(old_size <= num_taps),
      | %    new_size = old_size;
      | %else,
      | %    new_size = num_taps;
      | %end
      | 
      | %for n = 1:new_size, vec(n) = old_vec(n); end
      | %set_param(gcb, 'mult_spec', mat2str(vec));
      mask TypeOptions WindowType: bartlett | barthannwin | blackman | blackmanharris | bohamwin | chebwin | flattopwin | gausswin | hamming | hann | kaiser | nuttallwin | parzenwin | rectwin | tukeywin | triang | userwindow
      mask TypeOptions quantization: Truncate | Round  (unbiased: +/- Inf) | Round  (unbiased: Even Values)
      mask TypeOptions adder_imp: Behavioral | Fabric | DSP48
  pfb_fir_real3 : Subsystem  Tag=casper:pfb_fir_real  AncestorBlock=casper_library_pfbs/pfb_fir_real  mask(pfb_fir_real){PFBSize=2, TotalTaps=4, WindowType=hamming, n_inputs=0, MakeBiplex=off, BitWidthIn=8, BitWidthOut=18, CoeffBitWidth=18, CoeffDistMem=off, add_latency=1, mult_latency=2, bram_latency=2, fan_latency=1, conv_latency=1, quantization=Round  (unbiased: Even Values), fwidth=1, mult_spec=2, adder_folding=on, adder_imp=Fabric, coeffs_share=off}
      mask prompts: PFBSize "Size of PFB: (2^? pnts)"; TotalTaps "Total Number of Taps:"; WindowType "Windowing Function:"; n_inputs "Number of Simultaneous Inputs: (2^?)"; MakeBiplex "Make Biplex?"; BitWidthIn "Input Bitwidth:"; BitWidthOut "Output Bitwidth:"; CoeffBitWidth "Coefficient Bitwidth:"; CoeffDistMem "Use Distributed Memory for Coeffs"; add_latency "Add Latency"; mult_latency "Mult Latency"; bram_latency "BRAM Latency"; fan_latency "Fanout latency"; conv_latency "Convert latency"; quantization "Quantization Behavior"; fwidth "Bin Width Scaling (normal=1)"; mult_spec "Multiplier specification (0=core, 1=embedded, 2=behavioural) (left=1st tap, or just one value)"; adder_folding "Fold adders into DSPs"; adder_imp "Adder implementation"; coeffs_share "Share coefficients between polarisations (use less BRAM)?"
      mask help:
      | Fold adders into DSPs: Causes adders to be absorbed into DSP blocks (supported in Virtex5)
      | Adder implementation: Cores using Fabric or DSP48 or behavioral HDL
      mask init: same as adc16_dbf_4fft/pfb_single_channel/pfb_fir_real1
      settings: AttributesFormatString=taps=4, add_latency=1
      mask Help: eval('xlWeb(''http://casper.berkeley.edu/wiki/Pfb_fir_real'')')
      mask Callback TotalTaps:
      | %num_taps = eval(get_param(gcb, 'TotalTaps'));
      | %old_vec = eval(get_param(gcb, 'mult_spec'));=-0l
      | 
      | %vec = 2.*ones(1,num_taps);
      | %old_size = length(old_vec);
      | 
      | %if(old_size <= num_taps),
      | %    new_size = old_size;
      | %else,
      | %    new_size = num_taps;
      | %end
      | 
      | %for n = 1:new_size, vec(n) = old_vec(n); end
      | %set_param(gcb, 'mult_spec', mat2str(vec));
      mask TypeOptions WindowType: bartlett | barthannwin | blackman | blackmanharris | bohamwin | chebwin | flattopwin | gausswin | hamming | hann | kaiser | nuttallwin | parzenwin | rectwin | tukeywin | triang | userwindow
      mask TypeOptions quantization: Truncate | Round  (unbiased: +/- Inf) | Round  (unbiased: Even Values)
      mask TypeOptions adder_imp: Behavioral | Fabric | DSP48
  pfb_fir_real4 : Subsystem  Tag=casper:pfb_fir_real  AncestorBlock=casper_library_pfbs/pfb_fir_real  mask(pfb_fir_real){PFBSize=2, TotalTaps=4, WindowType=hamming, n_inputs=0, MakeBiplex=off, BitWidthIn=8, BitWidthOut=18, CoeffBitWidth=18, CoeffDistMem=off, add_latency=1, mult_latency=2, bram_latency=2, fan_latency=1, conv_latency=1, quantization=Round  (unbiased: Even Values), fwidth=1, mult_spec=2, adder_folding=on, adder_imp=Fabric, coeffs_share=off}
      mask prompts: PFBSize "Size of PFB: (2^? pnts)"; TotalTaps "Total Number of Taps:"; WindowType "Windowing Function:"; n_inputs "Number of Simultaneous Inputs: (2^?)"; MakeBiplex "Make Biplex?"; BitWidthIn "Input Bitwidth:"; BitWidthOut "Output Bitwidth:"; CoeffBitWidth "Coefficient Bitwidth:"; CoeffDistMem "Use Distributed Memory for Coeffs"; add_latency "Add Latency"; mult_latency "Mult Latency"; bram_latency "BRAM Latency"; fan_latency "Fanout latency"; conv_latency "Convert latency"; quantization "Quantization Behavior"; fwidth "Bin Width Scaling (normal=1)"; mult_spec "Multiplier specification (0=core, 1=embedded, 2=behavioural) (left=1st tap, or just one value)"; adder_folding "Fold adders into DSPs"; adder_imp "Adder implementation"; coeffs_share "Share coefficients between polarisations (use less BRAM)?"
      mask help:
      | Fold adders into DSPs: Causes adders to be absorbed into DSP blocks (supported in Virtex5)
      | Adder implementation: Cores using Fabric or DSP48 or behavioral HDL
      mask init: same as adc16_dbf_4fft/pfb_single_channel/pfb_fir_real1
      settings: AttributesFormatString=taps=4, add_latency=1
      mask Help: eval('xlWeb(''http://casper.berkeley.edu/wiki/Pfb_fir_real'')')
      mask Callback TotalTaps:
      | %num_taps = eval(get_param(gcb, 'TotalTaps'));
      | %old_vec = eval(get_param(gcb, 'mult_spec'));=-0l
      | 
      | %vec = 2.*ones(1,num_taps);
      | %old_size = length(old_vec);
      | 
      | %if(old_size <= num_taps),
      | %    new_size = old_size;
      | %else,
      | %    new_size = num_taps;
      | %end
      | 
      | %for n = 1:new_size, vec(n) = old_vec(n); end
      | %set_param(gcb, 'mult_spec', mat2str(vec));
      mask TypeOptions WindowType: bartlett | barthannwin | blackman | blackmanharris | bohamwin | chebwin | flattopwin | gausswin | hamming | hann | kaiser | nuttallwin | parzenwin | rectwin | tukeywin | triang | userwindow
      mask TypeOptions quantization: Truncate | Round  (unbiased: +/- Inf) | Round  (unbiased: Even Values)
      mask TypeOptions adder_imp: Behavioral | Fabric | DSP48
  sync_out : Outport
  pol1_out : Outport  Port=2
  pol2_out : Outport  Port=3
  pol3_out : Outport  Port=4
  pol4_out : Outport  Port=5
  wires:
  pfb_fir_real4/1(sync_out) -> Terminator2/1
  pfb_fir_real3/1(sync_out) -> Terminator1/1
  pfb_fir_real2/1(sync_out) -> Terminator/1
  pfb_fir_real1/1(sync_out) -> sync_out/1
  pfb_fir_real2/2(pol1_out1) -> pol2_out/1
  pol4_in/1 -> pfb_fir_real4/2(pol1_in1)
  pol1_in/1 -> pfb_fir_real1/2(pol1_in1)
  pfb_fir_real4/2(pol1_out1) -> pol4_out/1
  pfb_fir_real3/2(pol1_out1) -> pol3_out/1
  sync/1 -> pfb_fir_real1/1(sync), pfb_fir_real2/1(sync), pfb_fir_real3/1(sync), pfb_fir_real4/1(sync)
  pfb_fir_real1/2(pol1_out1) -> pol1_out/1
  pol3_in/1 -> pfb_fir_real3/2(pol1_in1)
  pol2_in/1 -> pfb_fir_real2/2(pol1_in1)
